simulink model "NGGenset_Test_System"  (Simulink 8.1)
settings: Solver=ode3  SolverMode=SingleTasking  StartTime=0.0  StopTime=150  FixedStep=Ts  RelTol=1e-3
PostLoadFcn:
  | Ts=50e-6;
InitFcn:
  | Ts=50e-6;
undefined symbols (not defined in the file): another_event_name, DiscIntNeverNeededParam, fdesignblkfcn, gcbh, Gen_900kW_external_control, HIL_GenSet, Left, my_event_name, ph, type, V
libraries: powerlib x47, simulink x40, powerlib_extras x28, rtio_opalrt_common x21, dspsigops x7, breakers_1ph_3ph x7, rtio_generic_modbus x7, simulink_extras x6, cables_lib x5, rteventslib x4, rtlab x3, discretizing x2
(part 4 of 5)

== system NGGenset_Test_System/SM_Master/Generator/Woodward Outputs/TSDIO - Gr3 ==
  TSDout : Inport
  Bus Creator : BusCreator  Inputs=16
  Bus Creator1 : BusCreator  Inputs=16
  Bus Creator2 : BusCreator  Inputs=2
  Bus Selector : BusSelector  OutputSignals=16 TSDOUT GR3.states.CH16-23.states 17,16 TSDOUT GR3.times CH16-23.times17,16 TSDOUT GR3.states.CH16-23.states 18,16 TSDOUT GR3.times CH16-23.times18,16 TSDOUT GR3.states.CH16-23.states 19,16 TSDOUT GR3.times CH16-23.times19,16 TSDOUT GR3.states.CH16-23.states 20,16 TSDOUT GR3.times CH16-23.times20,16 TSDOUT GR3.states.CH16-23.states 21,16 TSDOUT GR3.times CH16-23.times21,16 TSDOUT GR3.states.CH16-23.states 22,16 TSDOUT GR3.times CH16-23.times22,16 TSDOUT GR3.states.CH16-23.states 23,16 TSDOUT GR3.times CH16-23.times23,16 TSDOUT GR3.states.CH16-23.states 24,16 TSDOUT GR3.times CH16-23.times24
  Bus Selector1 : BusSelector  OutputSignals=16 TSDOUT GR3.states.CH24-31.states 25,16 TSDOUT GR3.times CH24-31.times25,16 TSDOUT GR3.states.CH24-31.states 26,16 TSDOUT GR3.times CH24-31.times26,16 TSDOUT GR3.states.CH24-31.states 27,16 TSDOUT GR3.times CH24-31.times27,16 TSDOUT GR3.states.CH24-31.states 28,16 TSDOUT GR3.times CH24-31.times28,16 TSDOUT GR3.states.CH24-31.states 29,16 TSDOUT GR3.times CH24-31.times29,16 TSDOUT GR3.states.CH24-31.states 30,16 TSDOUT GR3.times CH24-31.times30,16 TSDOUT GR3.states.CH24-31.states 31,16 TSDOUT GR3.times CH24-31.times31,16 TSDOUT GR3.states.CH24-31.states 32,16 TSDOUT GR3.times CH24-31.times32
  EventDetector : rtio_opalrt_common/EventDetector  CtrlName='OpCtrl'  portNb=7  FcnNos=Slot 3 Module A Subsection 3  size=32  maxcount=8  nbChannels=8  width=4  timeUnit=Time ratio  sampleTime=0  numwidth=4
      settings: AttributesFormatString=%<CtrlName>
  EventDetector1 : rtio_opalrt_common/EventDetector  CtrlName='OpCtrl'  portNb=8  FcnNos=Slot 3 Module A Subsection 4  size=32  maxcount=8  nbChannels=8  width=4  timeUnit=Time ratio  sampleTime=0  numwidth=4
      settings: AttributesFormatString=%<CtrlName>
  EventGenerator : rtio_opalrt_common/EventGenerator  CtrlName='OpCtrl'  portNb=7  FcnNos=Slot 3 Module B Subsection 3  size=32  count=8  nbChannels=8  width=4  timeUnit=Time ratio  numwidth=4
      settings: AttributesFormatString=%<CtrlName>
  EventGenerator1 : rtio_opalrt_common/EventGenerator  CtrlName='OpCtrl'  portNb=8  FcnNos=Slot 3 Module B Subsection 4  size=32  count=8  nbChannels=8  width=4  timeUnit=Time ratio  numwidth=4
      settings: AttributesFormatString=%<CtrlName>
  Terminator{,1..3} (4 alike) : Terminator
  TSDin : Outport
  wires:
  TSDout/1 -> Bus Selector/1, Bus Selector1/1
  Bus Selector/16 -> EventGenerator/16  "<times24>"
  Bus Selector/15 -> EventGenerator/15  "<states 24>"
  Bus Selector/14 -> EventGenerator/14  "<times23>"
  Bus Selector/13 -> EventGenerator/13  "<states 23>"
  Bus Selector/12 -> EventGenerator/12  "<times22>"
  Bus Selector/11 -> EventGenerator/11  "<states 22>"
  Bus Selector/10 -> EventGenerator/10  "<times21>"
  Bus Selector/9 -> EventGenerator/9  "<states 21>"
  Bus Selector/8 -> EventGenerator/8  "<times20>"
  Bus Selector/7 -> EventGenerator/7  "<states 20>"
  Bus Selector/6 -> EventGenerator/6  "<times19>"
  Bus Selector/5 -> EventGenerator/5  "<states 19>"
  Bus Selector/4 -> EventGenerator/4  "<times18>"
  Bus Selector/3 -> EventGenerator/3  "<states 18>"
  Bus Selector/2 -> EventGenerator/2  "<times17>"
  Bus Selector/1 -> EventGenerator/1  "<states 17>"
  EventGenerator/1 -> Terminator/1
  EventDetector/16 -> Bus Creator/16  "times8"
  EventDetector/15 -> Bus Creator/15  "states8"
  EventDetector/14 -> Bus Creator/14  "times7"
  EventDetector/13 -> Bus Creator/13  "states7"
  EventDetector/12 -> Bus Creator/12  "times6"
  EventDetector/11 -> Bus Creator/11  "states6"
  EventDetector/10 -> Bus Creator/10  "times5"
  EventDetector/9 -> Bus Creator/9  "states5"
  EventDetector/8 -> Bus Creator/8  "times4"
  EventDetector/7 -> Bus Creator/7  "states4"
  EventDetector/6 -> Bus Creator/6  "times3"
  EventDetector/5 -> Bus Creator/5  "states3"
  EventDetector/4 -> Bus Creator/4  "times2"
  EventDetector/3 -> Bus Creator/3  "states2"
  EventDetector/2 -> Bus Creator/2  "times1"
  EventDetector/1 -> Bus Creator/1  "states1"
  EventDetector/17 -> Terminator1/1
  EventGenerator1/1 -> Terminator2/1
  Bus Selector1/1 -> EventGenerator1/1  "<states 25>"
  Bus Selector1/2 -> EventGenerator1/2  "<times25>"
  Bus Selector1/3 -> EventGenerator1/3  "<states 26>"
  Bus Selector1/4 -> EventGenerator1/4  "<times26>"
  Bus Selector1/5 -> EventGenerator1/5  "<states 27>"
  Bus Selector1/6 -> EventGenerator1/6  "<times27>"
  Bus Selector1/7 -> EventGenerator1/7  "<states 28>"
  Bus Selector1/8 -> EventGenerator1/8  "<times28>"
  Bus Selector1/9 -> EventGenerator1/9  "<states 29>"
  Bus Selector1/10 -> EventGenerator1/10  "<times29>"
  Bus Selector1/11 -> EventGenerator1/11  "<states 30>"
  Bus Selector1/12 -> EventGenerator1/12  "<times30>"
  Bus Selector1/13 -> EventGenerator1/13  "<states 31>"
  Bus Selector1/14 -> EventGenerator1/14  "<times31>"
  Bus Selector1/15 -> EventGenerator1/15  "<states 32>"
  Bus Selector1/16 -> EventGenerator1/16  "<times32>"
  Bus Creator1/1 -> Bus Creator2/2  "CH24-31"
  EventDetector1/16 -> Bus Creator1/16  "times6"
  EventDetector1/15 -> Bus Creator1/15  "states6"
  EventDetector1/14 -> Bus Creator1/14  "times5"
  EventDetector1/13 -> Bus Creator1/13  "states5"
  EventDetector1/12 -> Bus Creator1/12  "times4"
  EventDetector1/11 -> Bus Creator1/11  "states4"
  EventDetector1/10 -> Bus Creator1/10  "times3"
  EventDetector1/9 -> Bus Creator1/9  "states3"
  EventDetector1/8 -> Bus Creator1/8  "times2"
  EventDetector1/7 -> Bus Creator1/7  "states2"
  EventDetector1/6 -> Bus Creator1/6  "times1"
  EventDetector1/5 -> Bus Creator1/5  "states1"
  EventDetector1/4 -> Bus Creator1/4  "times2"
  EventDetector1/3 -> Bus Creator1/3  "states2"
  EventDetector1/2 -> Bus Creator1/2  "times1"
  EventDetector1/1 -> Bus Creator1/1  "states1"
  EventDetector1/17 -> Terminator3/1  "states7"
  Bus Creator/1 -> Bus Creator2/1  "CH16-23"
  Bus Creator2/1 -> TSDin/1  "TSDIN"

== system NGGenset_Test_System/SM_Master/Generator/Woodward Outputs/Woodward Primary Inputs ==
  Bias-ctrl : Inport
  Bus Creator : BusCreator
  Bus Creator1 : BusCreator
  Constant{,5,10..11} (4 alike) : Constant  Value=1.00
  Constant{1,3..4,6,8..9} (6 alike) : Constant  Value=0
  Constant2 : Constant  Value=20
  Constant7 : Constant  Value=20
  Demux1 : Demux  Outputs=16
  Divide{,1..3} (4 alike) : Product  Inputs=*/
  GR1 B AIN (CH00-15) : Subsystem
  Lowpass Filter : Subsystem  DialogController=fdesignblkfcn  DialogControllerArgs=DataTag4  InitFcn=fdesignblkfcn(gcbh, {'InitFcn'});  mask(Lowpass Filter){}
      mask help: Design a lowpass filter
      settings: CopyFcn=fdesignblkfcn(gcbh, {'CopyFcn'});
      mask Help: helpview(mapfilelocation('dsp'), 'dsplowpassfilter');
      mask Display: disp('Lowpass')
  Lowpass Filter1 : Subsystem  DialogController=fdesignblkfcn  DialogControllerArgs=DataTag6  InitFcn=fdesignblkfcn(gcbh, {'InitFcn'});  mask(Lowpass Filter){}
      mask help: Design a lowpass filter
      settings: CopyFcn=fdesignblkfcn(gcbh, {'CopyFcn'});
      mask Help: helpview(mapfilelocation('dsp'), 'dsplowpassfilter');
      mask Display: disp('Lowpass')
  Lowpass Filter2 : Subsystem  DialogController=fdesignblkfcn  DialogControllerArgs=DataTag8  InitFcn=fdesignblkfcn(gcbh, {'InitFcn'});  mask(Lowpass Filter){}
      mask help: Design a lowpass filter
      settings: CopyFcn=fdesignblkfcn(gcbh, {'CopyFcn'});
      mask Help: helpview(mapfilelocation('dsp'), 'dsplowpassfilter');
      mask Display: disp('Lowpass')
  Lowpass Filter3 : Subsystem  DialogController=fdesignblkfcn  DialogControllerArgs=DataTag10  InitFcn=fdesignblkfcn(gcbh, {'InitFcn'});  mask(Lowpass Filter){}
      mask help: Design a lowpass filter
      settings: CopyFcn=fdesignblkfcn(gcbh, {'CopyFcn'});
      mask Help: helpview(mapfilelocation('dsp'), 'dsplowpassfilter');
      mask Display: disp('Lowpass')
  Sum{,1..3} (4 alike) : Sum  Inputs=|+-
  Switch{,1..3} (4 alike) : Switch  Threshold=0.5
  Gen1 Gov and AVR : Outport
  Gen2 Gov and AVR : Outport  Port=2
  wires:
  GR1 B AIN (CH00-15)/1(Out1) -> [AINs_Gr1], Demux1/1
  Demux1/1 -> Divide/1
  Demux1/2 -> Divide1/1
  Constant2/1 -> Divide1/2, Divide/2
  Divide/1 -> Sum/1
  Divide1/1 -> Sum1/1
  Constant3/1 -> Sum/2
  Constant4/1 -> Sum1/2
  Sum/1 -> Lowpass Filter/1(In)
  Switch/1 -> Bus Creator/3  "Gen1 Gov"
  Switch1/1 -> Bus Creator/4  "Gen1 AVR"
  Sum1/1 -> Lowpass Filter1/1(In)
  Constant1/1 -> Switch/3, Switch1/3
  Bias-ctrl/1 -> Switch/2, Switch1/2, Switch2/2, Switch3/2
  Lowpass Filter/1(Out) -> Switch/1
  Lowpass Filter1/1(Out) -> Switch1/1
  Constant5/1 -> Bus Creator/2  "Gen1 Ref AVR"
  Constant/1 -> Bus Creator/1  "Gen1 Ref GOV"
  Demux1/3 -> Divide2/1
  Demux1/4 -> Divide3/1
  Constant7/1 -> Divide3/2, Divide2/2
  Divide2/1 -> Sum2/1
  Divide3/1 -> Sum3/1
  Constant8/1 -> Sum2/2
  Constant9/1 -> Sum3/2
  Sum2/1 -> Lowpass Filter2/1(In)
  Switch2/1 -> Bus Creator1/3  "Gen2 GOV"
  Switch3/1 -> Bus Creator1/4  "Gen2 AVR"
  Sum3/1 -> Lowpass Filter3/1(In)
  Constant6/1 -> Switch2/3, Switch3/3
  Lowpass Filter2/1(Out) -> Switch2/1
  Lowpass Filter3/1(Out) -> Switch3/1
  Constant11/1 -> Bus Creator1/2  "Gen2 Ref AVR"
  Constant10/1 -> Bus Creator1/1  "Gen2 Ref GOV"
  Bus Creator/1 -> Gen1 Gov and AVR/1
  Bus Creator1/1 -> Gen2 Gov and AVR/1

== system NGGenset_Test_System/SM_Master/MODBUS1/SEL_787_Relay/PQ_Calculator ==
  Vabc : Inport
  Iabc : Inport  Port=2
  3-phase  Instantaneous  Active & Reactive Power : powerlib_extras/Measurements/3-phase  Instantaneous  Active & Reactive Power
  Demux : Demux  Outputs=2
  Discrete  Mean value2 : powerlib_extras/Discrete Measurements/Discrete  Mean value  Freq=60  Vinit=0  Ts=Ts
  P : Outport
  Q : Outport  Port=2
  wires:
  3-phase  Instantaneous  Active & Reactive Power/1 -> Discrete  Mean value2/1
  Discrete  Mean value2/1 -> Demux/1
  Vabc/1 -> 3-phase  Instantaneous  Active & Reactive Power/1
  Iabc/1 -> 3-phase  Instantaneous  Active & Reactive Power/2
  Demux/1 -> P/1  "P"
  Demux/2 -> Q/1  "Q"

== system NGGenset_Test_System/SM_Master/MODBUS1/SEL_787_Relay/RMS_Calculator ==
  Signal : Inport
  Discrete  Mean value6 : powerlib_extras/Discrete Measurements/Discrete  Mean value  Freq=60  Vinit=0  Ts=Ts
  Product3 : Product  RndMeth=Zero
  Signed Sqrt : Sqrt  SaturateOnIntegerOverflow=on
  RMS_Signal : Outport
  wires:
  Signal/1 -> Product3/1, Product3/2
  Product3/1 -> Discrete  Mean value6/1
  Discrete  Mean value6/1 -> Signed Sqrt/1
  Signed Sqrt/1 -> RMS_Signal/1

== system NGGenset_Test_System/SM_Master/MODBUS1/SEL_787_Relay/RMS_Calculator1 ==
  Signal : Inport
  Discrete  Mean value6 : powerlib_extras/Discrete Measurements/Discrete  Mean value  Freq=60  Vinit=0  Ts=Ts
  Product3 : Product  RndMeth=Zero
  Signed Sqrt : Sqrt  SaturateOnIntegerOverflow=on
  RMS_Signal : Outport
  wires:
  Signal/1 -> Product3/1, Product3/2
  Product3/1 -> Discrete  Mean value6/1
  Discrete  Mean value6/1 -> Signed Sqrt/1
  Signed Sqrt/1 -> RMS_Signal/1

== system NGGenset_Test_System/SM_Master/MODBUS1/SEL_787_Relay/pf_Calculator ==
  P : Inport
  Q : Inport  Port=2
  Fcn : Fcn  Expr=u(1) / sqrt(u(1)^2 + u(2)^2)
  Fcn1 : Fcn  Expr=sqrt(u(1)^2 + u(2)^2)
  Mux : Mux  Inputs=2
  Mux1 : Mux  Inputs=2
  Scope : Scope
      settings: YMin=0.8475  YMax=0.875  SaveName=ScopeData2
  pf : Outport
  S : Outport  Port=2
  wires:
  Fcn1/1 -> S/1
  Mux1/1 -> Fcn1/1
  Fcn/1 -> Scope/1, pf/1
  Mux/1 -> Fcn/1
  P/1 -> Mux1/1, Mux/1
  Q/1 -> Mux1/2, Mux/2

== system NGGenset_Test_System/SM_Master/MODBUS10/SEL_787_Relay/PQ_Calculator ==
  Vabc : Inport
  Iabc : Inport  Port=2
  3-phase  Instantaneous  Active & Reactive Power : powerlib_extras/Measurements/3-phase  Instantaneous  Active & Reactive Power
  Demux : Demux  Outputs=2
  Discrete  Mean value2 : powerlib_extras/Discrete Measurements/Discrete  Mean value  Freq=60  Vinit=0  Ts=Ts
  P : Outport
  Q : Outport  Port=2
  wires:
  3-phase  Instantaneous  Active & Reactive Power/1 -> Discrete  Mean value2/1
  Discrete  Mean value2/1 -> Demux/1
  Vabc/1 -> 3-phase  Instantaneous  Active & Reactive Power/1
  Iabc/1 -> 3-phase  Instantaneous  Active & Reactive Power/2
  Demux/1 -> P/1  "P"
  Demux/2 -> Q/1  "Q"

== system NGGenset_Test_System/SM_Master/MODBUS10/SEL_787_Relay/RMS_Calculator ==
  Signal : Inport
  Discrete  Mean value6 : powerlib_extras/Discrete Measurements/Discrete  Mean value  Freq=60  Vinit=0  Ts=Ts
  Product3 : Product  RndMeth=Zero
  Signed Sqrt : Sqrt  SaturateOnIntegerOverflow=on
  RMS_Signal : Outport
  wires:
  Signal/1 -> Product3/1, Product3/2
  Product3/1 -> Discrete  Mean value6/1
  Discrete  Mean value6/1 -> Signed Sqrt/1
  Signed Sqrt/1 -> RMS_Signal/1

== system NGGenset_Test_System/SM_Master/MODBUS10/SEL_787_Relay/RMS_Calculator1 ==
  Signal : Inport
  Discrete  Mean value6 : powerlib_extras/Discrete Measurements/Discrete  Mean value  Freq=60  Vinit=0  Ts=Ts
  Product3 : Product  RndMeth=Zero
  Signed Sqrt : Sqrt  SaturateOnIntegerOverflow=on
  RMS_Signal : Outport
  wires:
  Signal/1 -> Product3/1, Product3/2
  Product3/1 -> Discrete  Mean value6/1
  Discrete  Mean value6/1 -> Signed Sqrt/1
  Signed Sqrt/1 -> RMS_Signal/1

== system NGGenset_Test_System/SM_Master/MODBUS10/SEL_787_Relay/pf_Calculator ==
  P : Inport
  Q : Inport  Port=2
  Fcn : Fcn  Expr=u(1) / sqrt(u(1)^2 + u(2)^2)
  Fcn1 : Fcn  Expr=sqrt(u(1)^2 + u(2)^2)
  Mux : Mux  Inputs=2
  Mux1 : Mux  Inputs=2
  Scope : Scope
      settings: YMin=0.8475  YMax=0.875  SaveName=ScopeData2
  pf : Outport
  S : Outport  Port=2
  wires:
  Fcn1/1 -> S/1
  Mux1/1 -> Fcn1/1
  Fcn/1 -> Scope/1, pf/1
  Mux/1 -> Fcn/1
  P/1 -> Mux1/1, Mux/1
  Q/1 -> Mux1/2, Mux/2

== system NGGenset_Test_System/SM_Master/MODBUS2/SEL_787_Relay/PQ_Calculator ==
  Vabc : Inport
  Iabc : Inport  Port=2
  3-phase  Instantaneous  Active & Reactive Power : powerlib_extras/Measurements/3-phase  Instantaneous  Active & Reactive Power
  Demux : Demux  Outputs=2
  Discrete  Mean value2 : powerlib_extras/Discrete Measurements/Discrete  Mean value  Freq=60  Vinit=0  Ts=Ts
  P : Outport
  Q : Outport  Port=2
  wires:
  3-phase  Instantaneous  Active & Reactive Power/1 -> Discrete  Mean value2/1
  Discrete  Mean value2/1 -> Demux/1
  Vabc/1 -> 3-phase  Instantaneous  Active & Reactive Power/1
  Iabc/1 -> 3-phase  Instantaneous  Active & Reactive Power/2
  Demux/1 -> P/1  "P"
  Demux/2 -> Q/1  "Q"

== system NGGenset_Test_System/SM_Master/MODBUS2/SEL_787_Relay/RMS_Calculator ==
  Signal : Inport
  Discrete  Mean value6 : powerlib_extras/Discrete Measurements/Discrete  Mean value  Freq=60  Vinit=0  Ts=Ts
  Product3 : Product  RndMeth=Zero
  Signed Sqrt : Sqrt  SaturateOnIntegerOverflow=on
  RMS_Signal : Outport
  wires:
  Signal/1 -> Product3/1, Product3/2
  Product3/1 -> Discrete  Mean value6/1
  Discrete  Mean value6/1 -> Signed Sqrt/1
  Signed Sqrt/1 -> RMS_Signal/1

== system NGGenset_Test_System/SM_Master/MODBUS2/SEL_787_Relay/RMS_Calculator1 ==
  Signal : Inport
  Discrete  Mean value6 : powerlib_extras/Discrete Measurements/Discrete  Mean value  Freq=60  Vinit=0  Ts=Ts
  Product3 : Product  RndMeth=Zero
  Signed Sqrt : Sqrt  SaturateOnIntegerOverflow=on
  RMS_Signal : Outport
  wires:
  Signal/1 -> Product3/1, Product3/2
  Product3/1 -> Discrete  Mean value6/1
  Discrete  Mean value6/1 -> Signed Sqrt/1
  Signed Sqrt/1 -> RMS_Signal/1

== system NGGenset_Test_System/SM_Master/MODBUS2/SEL_787_Relay/pf_Calculator ==
  P : Inport
  Q : Inport  Port=2
  Fcn : Fcn  Expr=u(1) / sqrt(u(1)^2 + u(2)^2)
  Fcn1 : Fcn  Expr=sqrt(u(1)^2 + u(2)^2)
  Mux : Mux  Inputs=2
  Mux1 : Mux  Inputs=2
  Scope : Scope
      settings: YMin=0.8475  YMax=0.875  SaveName=ScopeData2
  pf : Outport
  S : Outport  Port=2
  wires:
  Fcn1/1 -> S/1
  Mux1/1 -> Fcn1/1
  Fcn/1 -> Scope/1, pf/1
  Mux/1 -> Fcn/1
  P/1 -> Mux1/1, Mux/1
  Q/1 -> Mux1/2, Mux/2

== system NGGenset_Test_System/SM_Master/MODBUS4/SEL_787_Relay/PQ_Calculator ==
  Vabc : Inport
  Iabc : Inport  Port=2
  3-phase  Instantaneous  Active & Reactive Power : powerlib_extras/Measurements/3-phase  Instantaneous  Active & Reactive Power
  Demux : Demux  Outputs=2
  Discrete  Mean value2 : powerlib_extras/Discrete Measurements/Discrete  Mean value  Freq=60  Vinit=0  Ts=Ts
  P : Outport
  Q : Outport  Port=2
  wires:
  3-phase  Instantaneous  Active & Reactive Power/1 -> Discrete  Mean value2/1
  Discrete  Mean value2/1 -> Demux/1
  Vabc/1 -> 3-phase  Instantaneous  Active & Reactive Power/1
  Iabc/1 -> 3-phase  Instantaneous  Active & Reactive Power/2
  Demux/1 -> P/1  "P"
  Demux/2 -> Q/1  "Q"

== system NGGenset_Test_System/SM_Master/MODBUS4/SEL_787_Relay/RMS_Calculator ==
  Signal : Inport
  Discrete  Mean value6 : powerlib_extras/Discrete Measurements/Discrete  Mean value  Freq=60  Vinit=0  Ts=Ts
  Product3 : Product  RndMeth=Zero
  Signed Sqrt : Sqrt  SaturateOnIntegerOverflow=on
  RMS_Signal : Outport
  wires:
  Signal/1 -> Product3/1, Product3/2
  Product3/1 -> Discrete  Mean value6/1
  Discrete  Mean value6/1 -> Signed Sqrt/1
  Signed Sqrt/1 -> RMS_Signal/1

== system NGGenset_Test_System/SM_Master/MODBUS4/SEL_787_Relay/RMS_Calculator1 ==
  Signal : Inport
  Discrete  Mean value6 : powerlib_extras/Discrete Measurements/Discrete  Mean value  Freq=60  Vinit=0  Ts=Ts
  Product3 : Product  RndMeth=Zero
  Signed Sqrt : Sqrt  SaturateOnIntegerOverflow=on
  RMS_Signal : Outport
  wires:
  Signal/1 -> Product3/1, Product3/2
  Product3/1 -> Discrete  Mean value6/1
  Discrete  Mean value6/1 -> Signed Sqrt/1
  Signed Sqrt/1 -> RMS_Signal/1

== system NGGenset_Test_System/SM_Master/MODBUS4/SEL_787_Relay/pf_Calculator ==
  P : Inport
  Q : Inport  Port=2
  Fcn : Fcn  Expr=u(1) / sqrt(u(1)^2 + u(2)^2)
  Fcn1 : Fcn  Expr=sqrt(u(1)^2 + u(2)^2)
  Mux : Mux  Inputs=2
  Mux1 : Mux  Inputs=2
  Scope : Scope
      settings: YMin=0.8475  YMax=0.875  SaveName=ScopeData2
  pf : Outport
  S : Outport  Port=2
  wires:
  Fcn1/1 -> S/1
  Mux1/1 -> Fcn1/1
  Fcn/1 -> Scope/1, pf/1
  Mux/1 -> Fcn/1
  P/1 -> Mux1/1, Mux/1
  Q/1 -> Mux1/2, Mux/2

== system NGGenset_Test_System/SM_Master/MODBUS5/SEL_787_Relay/PQ_Calculator ==
  Vabc : Inport
  Iabc : Inport  Port=2
  3-phase  Instantaneous  Active & Reactive Power : powerlib_extras/Measurements/3-phase  Instantaneous  Active & Reactive Power
  Demux : Demux  Outputs=2
  Discrete  Mean value2 : powerlib_extras/Discrete Measurements/Discrete  Mean value  Freq=60  Vinit=0  Ts=Ts
  P : Outport
  Q : Outport  Port=2
  wires:
  3-phase  Instantaneous  Active & Reactive Power/1 -> Discrete  Mean value2/1
  Discrete  Mean value2/1 -> Demux/1
  Vabc/1 -> 3-phase  Instantaneous  Active & Reactive Power/1
  Iabc/1 -> 3-phase  Instantaneous  Active & Reactive Power/2
  Demux/1 -> P/1  "P"
  Demux/2 -> Q/1  "Q"

== system NGGenset_Test_System/SM_Master/MODBUS5/SEL_787_Relay/RMS_Calculator ==
  Signal : Inport
  Discrete  Mean value6 : powerlib_extras/Discrete Measurements/Discrete  Mean value  Freq=60  Vinit=0  Ts=Ts
  Product3 : Product  RndMeth=Zero
  Signed Sqrt : Sqrt  SaturateOnIntegerOverflow=on
  RMS_Signal : Outport
  wires:
  Signal/1 -> Product3/1, Product3/2
  Product3/1 -> Discrete  Mean value6/1
  Discrete  Mean value6/1 -> Signed Sqrt/1
  Signed Sqrt/1 -> RMS_Signal/1

== system NGGenset_Test_System/SM_Master/MODBUS5/SEL_787_Relay/RMS_Calculator1 ==
  Signal : Inport
  Discrete  Mean value6 : powerlib_extras/Discrete Measurements/Discrete  Mean value  Freq=60  Vinit=0  Ts=Ts
  Product3 : Product  RndMeth=Zero
  Signed Sqrt : Sqrt  SaturateOnIntegerOverflow=on
  RMS_Signal : Outport
  wires:
  Signal/1 -> Product3/1, Product3/2
  Product3/1 -> Discrete  Mean value6/1
  Discrete  Mean value6/1 -> Signed Sqrt/1
  Signed Sqrt/1 -> RMS_Signal/1

== system NGGenset_Test_System/SM_Master/MODBUS5/SEL_787_Relay/pf_Calculator ==
  P : Inport
  Q : Inport  Port=2
  Fcn : Fcn  Expr=u(1) / sqrt(u(1)^2 + u(2)^2)
  Fcn1 : Fcn  Expr=sqrt(u(1)^2 + u(2)^2)
  Mux : Mux  Inputs=2
  Mux1 : Mux  Inputs=2
  Scope : Scope
      settings: YMin=0.8475  YMax=0.875  SaveName=ScopeData2
  pf : Outport
  S : Outport  Port=2
  wires:
  Fcn1/1 -> S/1
  Mux1/1 -> Fcn1/1
  Fcn/1 -> Scope/1, pf/1
  Mux/1 -> Fcn/1
  P/1 -> Mux1/1, Mux/1
  Q/1 -> Mux1/2, Mux/2

== system NGGenset_Test_System/SM_Master/MODBUS6/SEL_787_Relay/PQ_Calculator ==
  Vabc : Inport
  Iabc : Inport  Port=2
  3-phase  Instantaneous  Active & Reactive Power : powerlib_extras/Measurements/3-phase  Instantaneous  Active & Reactive Power
  Demux : Demux  Outputs=2
  Discrete  Mean value2 : powerlib_extras/Discrete Measurements/Discrete  Mean value  Freq=60  Vinit=0  Ts=Ts
  P : Outport
  Q : Outport  Port=2
  wires:
  3-phase  Instantaneous  Active & Reactive Power/1 -> Discrete  Mean value2/1
  Discrete  Mean value2/1 -> Demux/1
  Vabc/1 -> 3-phase  Instantaneous  Active & Reactive Power/1
  Iabc/1 -> 3-phase  Instantaneous  Active & Reactive Power/2
  Demux/1 -> P/1  "P"
  Demux/2 -> Q/1  "Q"

== system NGGenset_Test_System/SM_Master/MODBUS6/SEL_787_Relay/RMS_Calculator ==
  Signal : Inport
  Discrete  Mean value6 : powerlib_extras/Discrete Measurements/Discrete  Mean value  Freq=60  Vinit=0  Ts=Ts
  Product3 : Product  RndMeth=Zero
  Signed Sqrt : Sqrt  SaturateOnIntegerOverflow=on
  RMS_Signal : Outport
  wires:
  Signal/1 -> Product3/1, Product3/2
  Product3/1 -> Discrete  Mean value6/1
  Discrete  Mean value6/1 -> Signed Sqrt/1
  Signed Sqrt/1 -> RMS_Signal/1

== system NGGenset_Test_System/SM_Master/MODBUS6/SEL_787_Relay/RMS_Calculator1 ==
  Signal : Inport
  Discrete  Mean value6 : powerlib_extras/Discrete Measurements/Discrete  Mean value  Freq=60  Vinit=0  Ts=Ts
  Product3 : Product  RndMeth=Zero
  Signed Sqrt : Sqrt  SaturateOnIntegerOverflow=on
  RMS_Signal : Outport
  wires:
  Signal/1 -> Product3/1, Product3/2
  Product3/1 -> Discrete  Mean value6/1
  Discrete  Mean value6/1 -> Signed Sqrt/1
  Signed Sqrt/1 -> RMS_Signal/1

== system NGGenset_Test_System/SM_Master/MODBUS6/SEL_787_Relay/pf_Calculator ==
  P : Inport
  Q : Inport  Port=2
  Fcn : Fcn  Expr=u(1) / sqrt(u(1)^2 + u(2)^2)
  Fcn1 : Fcn  Expr=sqrt(u(1)^2 + u(2)^2)
  Mux : Mux  Inputs=2
  Mux1 : Mux  Inputs=2
  Scope : Scope
      settings: YMin=0.8475  YMax=0.875  SaveName=ScopeData2
  pf : Outport
  S : Outport  Port=2
  wires:
  Fcn1/1 -> S/1
  Mux1/1 -> Fcn1/1
  Fcn/1 -> Scope/1, pf/1
  Mux/1 -> Fcn/1
  P/1 -> Mux1/1, Mux/1
  Q/1 -> Mux1/2, Mux/2

== system NGGenset_Test_System/SM_Master/MODBUS8/SEL_787_Relay/PQ_Calculator ==
  Vabc : Inport
  Iabc : Inport  Port=2
  3-phase  Instantaneous  Active & Reactive Power : powerlib_extras/Measurements/3-phase  Instantaneous  Active & Reactive Power
  Demux : Demux  Outputs=2
  Discrete  Mean value2 : powerlib_extras/Discrete Measurements/Discrete  Mean value  Freq=60  Vinit=0  Ts=Ts
  P : Outport
  Q : Outport  Port=2
  wires:
  3-phase  Instantaneous  Active & Reactive Power/1 -> Discrete  Mean value2/1
  Discrete  Mean value2/1 -> Demux/1
  Vabc/1 -> 3-phase  Instantaneous  Active & Reactive Power/1
  Iabc/1 -> 3-phase  Instantaneous  Active & Reactive Power/2
  Demux/1 -> P/1  "P"
  Demux/2 -> Q/1  "Q"

== system NGGenset_Test_System/SM_Master/MODBUS8/SEL_787_Relay/RMS_Calculator ==
  Signal : Inport
  Discrete  Mean value6 : powerlib_extras/Discrete Measurements/Discrete  Mean value  Freq=60  Vinit=0  Ts=Ts
  Product3 : Product  RndMeth=Zero
  Signed Sqrt : Sqrt  SaturateOnIntegerOverflow=on
  RMS_Signal : Outport
  wires:
  Signal/1 -> Product3/1, Product3/2
  Product3/1 -> Discrete  Mean value6/1
  Discrete  Mean value6/1 -> Signed Sqrt/1
  Signed Sqrt/1 -> RMS_Signal/1

== system NGGenset_Test_System/SM_Master/MODBUS8/SEL_787_Relay/RMS_Calculator1 ==
  Signal : Inport
  Discrete  Mean value6 : powerlib_extras/Discrete Measurements/Discrete  Mean value  Freq=60  Vinit=0  Ts=Ts
  Product3 : Product  RndMeth=Zero
  Signed Sqrt : Sqrt  SaturateOnIntegerOverflow=on
  RMS_Signal : Outport
  wires:
  Signal/1 -> Product3/1, Product3/2
  Product3/1 -> Discrete  Mean value6/1
  Discrete  Mean value6/1 -> Signed Sqrt/1
  Signed Sqrt/1 -> RMS_Signal/1

== system NGGenset_Test_System/SM_Master/MODBUS8/SEL_787_Relay/pf_Calculator ==
  P : Inport
  Q : Inport  Port=2
  Fcn : Fcn  Expr=u(1) / sqrt(u(1)^2 + u(2)^2)
  Fcn1 : Fcn  Expr=sqrt(u(1)^2 + u(2)^2)
  Mux : Mux  Inputs=2
  Mux1 : Mux  Inputs=2
  Scope : Scope
      settings: YMin=0.8475  YMax=0.875  SaveName=ScopeData2
  pf : Outport
  S : Outport  Port=2
  wires:
  Fcn1/1 -> S/1
  Mux1/1 -> Fcn1/1
  Fcn/1 -> Scope/1, pf/1
  Mux/1 -> Fcn/1
  P/1 -> Mux1/1, Mux/1
  Q/1 -> Mux1/2, Mux/2

== system NGGenset_Test_System/SC_Console/Woodward/16TSDIn/16 TSDOut GR3/Dout state ctrl/Dout_CH16_CH23 ==
  Bus Creator1 : BusCreator  Inputs=8
  Dout_CH{16..23} (8 alike) : Constant  Value=[1 0 1 0]
  Manual Switch{17..24} (8 alike) : ManualSwitch
  Zero_Dout_CH{16..23} (8 alike) : Constant  Value=[0 0 0 0]
  Dout_CH8_CH15 : Outport
  wires:
  Manual Switch24/1 -> Bus Creator1/8  "states 24"
  Manual Switch23/1 -> Bus Creator1/7  "states 23"
  Manual Switch22/1 -> Bus Creator1/6  "states 22"
  Manual Switch21/1 -> Bus Creator1/5  "states 21"
  Manual Switch20/1 -> Bus Creator1/4  "states 20"
  Manual Switch19/1 -> Bus Creator1/3  "states 19"
  Manual Switch18/1 -> Bus Creator1/2  "states 18"
  Manual Switch17/1 -> Bus Creator1/1  "states 17"
  Zero_Dout_CH23/1 -> Manual Switch24/2
  Dout_CH23/1 -> Manual Switch24/1
  Zero_Dout_CH22/1 -> Manual Switch23/2
  Dout_CH22/1 -> Manual Switch23/1
  Zero_Dout_CH21/1 -> Manual Switch22/2
  Dout_CH21/1 -> Manual Switch22/1
  Zero_Dout_CH20/1 -> Manual Switch21/2
  Dout_CH20/1 -> Manual Switch21/1
  Zero_Dout_CH19/1 -> Manual Switch20/2
  Dout_CH19/1 -> Manual Switch20/1
  Zero_Dout_CH18/1 -> Manual Switch19/2
  Dout_CH18/1 -> Manual Switch19/1
  Zero_Dout_CH17/1 -> Manual Switch18/2
  Dout_CH17/1 -> Manual Switch18/1
  Zero_Dout_CH16/1 -> Manual Switch17/2
  Dout_CH16/1 -> Manual Switch17/1
  Bus Creator1/1 -> Dout_CH8_CH15/1

== system NGGenset_Test_System/SC_Console/Woodward/16TSDIn/16 TSDOut GR3/Dout state ctrl/Dout_CH24_CH31 ==
  Bus Creator : BusCreator  Inputs=8
  Dout_CH{24..31} (8 alike) : Constant  Value=[1 0 1 0]
  Manual Switch{25..32} (8 alike) : ManualSwitch
  Zero_Dout_CH{24..31} (8 alike) : Constant  Value=[0 0 0 0]
  Dout_CH8_CH15 : Outport
  wires:
  Bus Creator/1 -> Dout_CH8_CH15/1
  Dout_CH24/1 -> Manual Switch25/1
  Zero_Dout_CH24/1 -> Manual Switch25/2
  Dout_CH25/1 -> Manual Switch26/1
  Zero_Dout_CH25/1 -> Manual Switch26/2
  Dout_CH26/1 -> Manual Switch27/1
  Zero_Dout_CH26/1 -> Manual Switch27/2
  Dout_CH27/1 -> Manual Switch28/1
  Zero_Dout_CH27/1 -> Manual Switch28/2
  Dout_CH28/1 -> Manual Switch29/1
  Zero_Dout_CH28/1 -> Manual Switch29/2
  Dout_CH29/1 -> Manual Switch30/1
  Zero_Dout_CH29/1 -> Manual Switch30/2
  Dout_CH30/1 -> Manual Switch31/1
  Zero_Dout_CH30/1 -> Manual Switch31/2
  Dout_CH31/1 -> Manual Switch32/1
  Zero_Dout_CH31/1 -> Manual Switch32/2
  Manual Switch25/1 -> Bus Creator/1  "states 25"
  Manual Switch26/1 -> Bus Creator/2  "states 26"
  Manual Switch27/1 -> Bus Creator/3  "states 27"
  Manual Switch28/1 -> Bus Creator/4  "states 28"
  Manual Switch29/1 -> Bus Creator/5  "states 29"
  Manual Switch30/1 -> Bus Creator/6  "states 30"
  Manual Switch31/1 -> Bus Creator/7  "states 31"
  Manual Switch32/1 -> Bus Creator/8  "states 32"

== system NGGenset_Test_System/SM_Master/Generator/GenSet_4MVA_copy1mva/4MVA Generator with  Primary Controllers/Diesel Engine Speed & Voltage Control fast ==
  note: originally ++
  note: originally ++
  note: These biases may need to
      | go to the references as opposed
      | to the measured signal.
  note: This is the device analog output of =-10Vdc to
      | the HIL Analog Input it should be scaled to 1 pu
  wref : Inport  SampleTime=Ts
  Vtref : Inport  Port=2  SampleTime=Ts
  Generator Enable : Inport  Port=3  SampleTime=Ts
  m : Inport  Port=4  SampleTime=Ts
  w_meas_Wood : Inport  Port=5  SampleTime=Ts
  V_meas_Wood : Inport  Port=6  SampleTime=Ts
  Woodward Enable : Inport  Port=7  SampleTime=Ts
  Bus Creator : BusCreator  Inputs=2
  Bus Creator1 : BusCreator  Inputs=2
  Bus Creator2 : BusCreator  Inputs=2
  Bus Selector : BusSelector  OutputSignals="Mechanical.Rotor speed  wm (pu)"
  Bus Selector1 : BusSelector  OutputSignals="dq0 components.Stator voltage  vd (pu),dq0 components.Stator voltage  vq (pu)"  OutputAsBus=on
  Bus to Vector : BusToVector
  Constant1 : Constant  Value=0
  Constant2 : Constant  Value=0
  Discrete PID Controller1 : simulink/Continuous/PID Controller  Controller=PID  TimeDomain=Discrete-time  SampleTime=-1  IntegratorMethod=Forward Euler  FilterMethod=Forward Euler  Form=Parallel  P=1  I=0  D=0  N=100  InitialConditionSource=internal  InitialConditionForIntegrator=0  InitialConditionForFilter=0  ExternalReset=either  LimitOutput=on  UpperSaturationLimit=5  LowerSaturationLimit=-5  LinearizeAsGain=off  AntiWindupMode=none  Kb=1  TrackingMode=off  Kt=1  PParamMin=[]  PParamMax=[]  IParamMin=[]  IParamMax=[]  DParamMin=[]  DParamMax=[]  NParamMin=[]  NParamMax=[]  KbParamMin=[]  KbParamMax=[]  KtParamMin=[]  KtParamMax=[]  POutMin=[]  POutMax=[]  IOutMin=[]  IOutMax=[]  DOutMin=[]  DOutMax=[]  NOutMin=[]  NOutMax=[]  KbOutMin=[]  KbOutMax=[]  KtOutMin=[]  KtOutMax=[]  IntegratorOutMin=[]  IntegratorOutMax=[]  FilterOutMin=[]  FilterOutMax=[]  SumOutMin=[]  SumOutMax=[]  SumI1OutMin=[]  SumI1OutMax=[]  SumI2OutMin=[]  SumI2OutMax=[]  SumI3OutMin=[]  SumI3OutMax=[]  SumDOutMin=[]  SumDOutMax=[]  SaturationOutMin=[]  SaturationOutMax=[]  IntegratorContinuousStateAttributes=''  IntegratorStateMustResolveToSignalObject=off  IntegratorRTWStateStorageClass=Auto  FilterContinuousStateAttributes=''  FilterStateMustResolveToSignalObject=off  FilterRTWStateStorageClass=Auto
  Excitation : Subsystem  mask(Excitation System){tr=20e-4, reg=[ 200 2e-3 ], exc=[ 1 0.00000001 ], tgr=[ 1e-12 1e-12 ], damp=[0 1e-12 ], sat=[], lim=[ 0 5 0 ], v0=[ 0 0 ]}
      mask prompts: tr "Low-pass filter time constant Tr:"; reg "Regulator gain and time constant [ Ka  Ta ]:"; exc "Exciter  [ Ke  Te ]:"; tgr "Transient gain reduction [ Tb  Tc ]:"; damp "Damping filter gain and time constant  [ Kf  Tf  ]:"; sat "Field saturation parameters [ A B ]:"; lim "Regulator output limits and gain [ Efmin  Efmax  Kp ]:"; v0 "Initial values of terminal voltage  and field voltage [ Vt0 Vf0 ] :"
      mask help:
      | Implements an IEEE type 1 synchronous machine voltage regulator combined
      | to an exciter.
      |
      | The output of the block is the field voltage vfd, in pu,  to be applied to the Vf
      | Simulink input of a Synchronous Machine block.
      |
      | Connect the Vd and Vq measurements signals of the Synchronous Machine block
      | (signals 9 and 10)  to  the Vd and Vq inputs of the Excitation System block.
      mask Help: helpview(psbhelp);
  Fcn1 : Fcn  Expr=sqrt(u(1)^2 + u(2)^2)
  GOVERNOR & DIESEL ENGINE1 : Subsystem  mask(Diesel Engine & Governor){K=10, Ta=[0.025 0.0009 0.00574], Tlim=[0 1.1], Td=0.024, Pm0=0.00005}
      mask prompts: K "Regulator gain K:"; Ta "Actuator time constants [T4 T5 T6] (s) :"; Tlim "Torque limits [Tmin Tmax] (pu) :"; Td "Engine time delay Td (s) :"; Pm0 "Initial value of mechanical power  Pm0 (pu) :"
      mask help:
      | This block implements a diesel engine and governor system:
      | 1st and 2nd inputs: Desired and actual speed (pu)
      | Output: Diesel engine mechanical power.Motor inertia should be combined with generator.
      |
      | Actuator transfer function :
      |      Ha= (1+T4.s) / [ (s (1+T5.s)(1+T6.s) ]
      | Motor :
      |      Time delay Td
      |
      | (See reference in Tutorial Session 5)
  Ground : Ground
  Scope : Scope
      settings: YMin=-5.5  YMax=5.5
  Sum : Sum  Inputs=|++
  Sum1 : Sum  Inputs=|++
  Switch1 : Switch  Threshold=0.5
  Switch2 : Switch  Threshold=0.5
  Pm : Outport
  Vf : Outport  Port=2
  Vt : Outport  Port=3
  w : Outport  Port=4
  Misc : Outport  Port=5
  wires:
  Sum/1 -> GOVERNOR & DIESEL ENGINE1/1(wref (pu))  "wms"
  wref/1 -> Sum/2
  Sum1/1 -> Excitation/1(vref)
  Vtref/1 -> Sum1/2
  Switch2/1 -> Bus Creator1/1, Sum1/1  "wood_AVR_bias"
  Constant1/1 -> Switch2/3
  Constant2/1 -> Switch1/3
  w_meas_Wood/1 -> Switch1/1
  Switch1/1 -> Bus Creator/1, Sum/1  "wood_Gov_bias"
  Woodward Enable/1 -> Switch2/2, Switch1/2
  Bus Creator2/1 -> Misc/1, Scope/1
  Discrete PID Controller1/1 -> Bus Creator2/2, Vf/1  "Vf_after"
  Excitation/1(Vf1) -> Bus Creator2/1, Discrete PID Controller1/1  "Vf_before"
  Bus Creator1/1 -> Vt/1
  Bus Creator/1 -> w/1
  Ground/1 -> Excitation/3(vstab)
  Fcn1/1 -> Excitation/2(v), Bus Creator1/2  "vms"
  V_meas_Wood/1 -> Switch2/1
  Bus Selector/1 -> GOVERNOR & DIESEL ENGINE1/2(w (pu)), Bus Creator/2  "<Rotor speed  wm (pu)>"
  m/1 -> Bus Selector1/1, Bus Selector/1
  Bus Selector1/1 -> Bus to Vector/1
  Bus to Vector/1 -> Fcn1/1
  Generator Enable/1 -> Discrete PID Controller1/2, GOVERNOR & DIESEL ENGINE1/3(Reset)
  GOVERNOR & DIESEL ENGINE1/1(Pmec (pu)) -> Pm/1  "Pmec_gov"

== system NGGenset_Test_System/SM_Master/Generator/GenSet_4MVA_copy1mva/Simulated Generator Controller 3.5 MW/PQ control ==
  P_ref (pu) : Inport
  P (pu) : Inport  Port=2
  Q_ref (pu) : Inport  Port=3
  Q (pu) : Inport  Port=4
  Discrete PID Controller : simulink/Continuous/PID Controller  Controller=PID  TimeDomain=Discrete-time  SampleTime=-1  IntegratorMethod=Forward Euler  FilterMethod=Forward Euler  Form=Parallel  P=0.025  I=1  D=0  N=10  InitialConditionSource=internal  InitialConditionForIntegrator=0  InitialConditionForFilter=0  ExternalReset=none  LimitOutput=on  UpperSaturationLimit=1.15  LowerSaturationLimit=0.85  LinearizeAsGain=off  AntiWindupMode=back-calculation  Kb=1  TrackingMode=off  Kt=1  PParamMin=[]  PParamMax=[]  IParamMin=[]  IParamMax=[]  DParamMin=[]  DParamMax=[]  NParamMin=[]  NParamMax=[]  KbParamMin=[]  KbParamMax=[]  KtParamMin=[]  KtParamMax=[]  POutMin=[]  POutMax=[]  IOutMin=[]  IOutMax=[]  DOutMin=[]  DOutMax=[]  NOutMin=[]  NOutMax=[]  KbOutMin=[]  KbOutMax=[]  KtOutMin=[]  KtOutMax=[]  IntegratorOutMin=[]  IntegratorOutMax=[]  FilterOutMin=[]  FilterOutMax=[]  SumOutMin=[]  SumOutMax=[]  SumI1OutMin=[]  SumI1OutMax=[]  SumI2OutMin=[]  SumI2OutMax=[]  SumI3OutMin=[]  SumI3OutMax=[]  SumDOutMin=[]  SumDOutMax=[]  SaturationOutMin=[]  SaturationOutMax=[]  IntegratorContinuousStateAttributes=''  IntegratorStateMustResolveToSignalObject=off  IntegratorRTWStateStorageClass=Auto  FilterContinuousStateAttributes=''  FilterStateMustResolveToSignalObject=off  FilterRTWStateStorageClass=Auto
  Discrete PID Controller1 : simulink/Continuous/PID Controller  Controller=PID  TimeDomain=Discrete-time  SampleTime=-1  IntegratorMethod=Forward Euler  FilterMethod=Forward Euler  Form=Parallel  P=0.2  I=1.5  D=0  N=10  InitialConditionSource=internal  InitialConditionForIntegrator=0  InitialConditionForFilter=0  ExternalReset=none  LimitOutput=on  UpperSaturationLimit=1.15  LowerSaturationLimit=0.85  LinearizeAsGain=off  AntiWindupMode=back-calculation  Kb=1  TrackingMode=off  Kt=1  PParamMin=[]  PParamMax=[]  IParamMin=[]  IParamMax=[]  DParamMin=[]  DParamMax=[]  NParamMin=[]  NParamMax=[]  KbParamMin=[]  KbParamMax=[]  KtParamMin=[]  KtParamMax=[]  POutMin=[]  POutMax=[]  IOutMin=[]  IOutMax=[]  DOutMin=[]  DOutMax=[]  NOutMin=[]  NOutMax=[]  KbOutMin=[]  KbOutMax=[]  KtOutMin=[]  KtOutMax=[]  IntegratorOutMin=[]  IntegratorOutMax=[]  FilterOutMin=[]  FilterOutMax=[]  SumOutMin=[]  SumOutMax=[]  SumI1OutMin=[]  SumI1OutMax=[]  SumI2OutMin=[]  SumI2OutMax=[]  SumI3OutMin=[]  SumI3OutMax=[]  SumDOutMin=[]  SumDOutMax=[]  SaturationOutMin=[]  SaturationOutMax=[]  IntegratorContinuousStateAttributes=''  IntegratorStateMustResolveToSignalObject=off  IntegratorRTWStateStorageClass=Auto  FilterContinuousStateAttributes=''  FilterStateMustResolveToSignalObject=off  FilterRTWStateStorageClass=Auto
  Sum : Sum  Inputs=|-+
  Sum1 : Sum  Inputs=|-+
  w_ref (pu) : Outport
  V_ref (pu) : Outport  Port=2
  wires:
  Q_ref (pu)/1 -> Sum1/2  "ref"
  Discrete PID Controller1/1 -> V_ref (pu)/1  "v"
  Q (pu)/1 -> Sum1/1  "pu"
  Sum1/1 -> Discrete PID Controller1/1  "dq"
  P_ref (pu)/1 -> Sum/2
  Discrete PID Controller/1 -> w_ref (pu)/1
  P (pu)/1 -> Sum/1
  Sum/1 -> Discrete PID Controller/1

== system NGGenset_Test_System/SM_Master/Generator/GenSet_4MVA_copy1mva/Simulated Generator Controller 3.5 MW/PV control ==
  P_ref (pu) : Inport
  P (pu) : Inport  Port=2
  Discrete PID Controller : simulink/Continuous/PID Controller  Controller=PID  TimeDomain=Discrete-time  SampleTime=-1  IntegratorMethod=Forward Euler  FilterMethod=Forward Euler  Form=Parallel  P=0.025  I=1  D=0  N=10  InitialConditionSource=internal  InitialConditionForIntegrator=0  InitialConditionForFilter=0  ExternalReset=none  LimitOutput=on  UpperSaturationLimit=1.15  LowerSaturationLimit=0.85  LinearizeAsGain=off  AntiWindupMode=back-calculation  Kb=1  TrackingMode=off  Kt=1  PParamMin=[]  PParamMax=[]  IParamMin=[]  IParamMax=[]  DParamMin=[]  DParamMax=[]  NParamMin=[]  NParamMax=[]  KbParamMin=[]  KbParamMax=[]  KtParamMin=[]  KtParamMax=[]  POutMin=[]  POutMax=[]  IOutMin=[]  IOutMax=[]  DOutMin=[]  DOutMax=[]  NOutMin=[]  NOutMax=[]  KbOutMin=[]  KbOutMax=[]  KtOutMin=[]  KtOutMax=[]  IntegratorOutMin=[]  IntegratorOutMax=[]  FilterOutMin=[]  FilterOutMax=[]  SumOutMin=[]  SumOutMax=[]  SumI1OutMin=[]  SumI1OutMax=[]  SumI2OutMin=[]  SumI2OutMax=[]  SumI3OutMin=[]  SumI3OutMax=[]  SumDOutMin=[]  SumDOutMax=[]  SaturationOutMin=[]  SaturationOutMax=[]  IntegratorContinuousStateAttributes=''  IntegratorStateMustResolveToSignalObject=off  IntegratorRTWStateStorageClass=Auto  FilterContinuousStateAttributes=''  FilterStateMustResolveToSignalObject=off  FilterRTWStateStorageClass=Auto
  Sum : Sum  Inputs=|-+
  w_ref (pu) : Outport
  wires:
  Sum/1 -> Discrete PID Controller/1
  P (pu)/1 -> Sum/1
  Discrete PID Controller/1 -> w_ref (pu)/1
  P_ref (pu)/1 -> Sum/2

== system NGGenset_Test_System/SM_Master/Generator/NG GenSet_3.5MVA_09212015/3.5MVA Generator with  Primary Controllers1/NG Engine Speed & Voltage Control fast ==
  note: originally ++
  note: originally ++
  note: These biases may need to
      | go to the references as opposed
      | to the measured signal.
  note: This is the device analog output of =-10Vdc to
      | the HIL Analog Input it should be scaled to 1 pu
  wref : Inport  SampleTime=Ts
  Vtref : Inport  Port=2  SampleTime=Ts
  Generator Enable : Inport  Port=3  SampleTime=Ts
  m : Inport  Port=4  SampleTime=Ts
  w_meas_Wood : Inport  Port=5  SampleTime=Ts
  V_meas_Wood : Inport  Port=6  SampleTime=Ts
  Woodward Enable : Inport  Port=7  SampleTime=Ts
  Bus Creator : BusCreator  Inputs=2
  Bus Creator1 : BusCreator  Inputs=2
  Bus Creator2 : BusCreator  Inputs=2
  Bus Selector : BusSelector  OutputSignals="Mechanical.Rotor speed  wm (pu)"
  Bus Selector1 : BusSelector  OutputSignals="dq0 components.Stator voltage  vd (pu),dq0 components.Stator voltage  vq (pu)"  OutputAsBus=on
  Bus to Vector : BusToVector
  Constant1 : Constant  Value=0
  Constant2 : Constant  Value=0
  Discrete PID Controller1 : simulink/Continuous/PID Controller  Controller=PID  TimeDomain=Discrete-time  SampleTime=-1  IntegratorMethod=Forward Euler  FilterMethod=Forward Euler  Form=Parallel  P=1  I=0  D=0  N=100  InitialConditionSource=internal  InitialConditionForIntegrator=0  InitialConditionForFilter=0  ExternalReset=either  LimitOutput=on  UpperSaturationLimit=5  LowerSaturationLimit=-5  LinearizeAsGain=off  AntiWindupMode=none  Kb=1  TrackingMode=off  Kt=1  PParamMin=[]  PParamMax=[]  IParamMin=[]  IParamMax=[]  DParamMin=[]  DParamMax=[]  NParamMin=[]  NParamMax=[]  KbParamMin=[]  KbParamMax=[]  KtParamMin=[]  KtParamMax=[]  POutMin=[]  POutMax=[]  IOutMin=[]  IOutMax=[]  DOutMin=[]  DOutMax=[]  NOutMin=[]  NOutMax=[]  KbOutMin=[]  KbOutMax=[]  KtOutMin=[]  KtOutMax=[]  IntegratorOutMin=[]  IntegratorOutMax=[]  FilterOutMin=[]  FilterOutMax=[]  SumOutMin=[]  SumOutMax=[]  SumI1OutMin=[]  SumI1OutMax=[]  SumI2OutMin=[]  SumI2OutMax=[]  SumI3OutMin=[]  SumI3OutMax=[]  SumDOutMin=[]  SumDOutMax=[]  SaturationOutMin=[]  SaturationOutMax=[]  IntegratorContinuousStateAttributes=''  IntegratorStateMustResolveToSignalObject=off  IntegratorRTWStateStorageClass=Auto  FilterContinuousStateAttributes=''  FilterStateMustResolveToSignalObject=off  FilterRTWStateStorageClass=Auto
  Excitation : Subsystem  mask(Excitation System){tr=20e-4, reg=[ 200 2e-3 ], exc=[ 1 0.00000001 ], tgr=[ 1e-12 1e-12 ], damp=[0 1e-12 ], sat=[], lim=[ 0 5 0 ], v0=[ 0 0 ]}
      mask prompts: tr "Low-pass filter time constant Tr:"; reg "Regulator gain and time constant [ Ka  Ta ]:"; exc "Exciter  [ Ke  Te ]:"; tgr "Transient gain reduction [ Tb  Tc ]:"; damp "Damping filter gain and time constant  [ Kf  Tf  ]:"; sat "Field saturation parameters [ A B ]:"; lim "Regulator output limits and gain [ Efmin  Efmax  Kp ]:"; v0 "Initial values of terminal voltage  and field voltage [ Vt0 Vf0 ] :"
      mask help:
      | Implements an IEEE type 1 synchronous machine voltage regulator combined
      | to an exciter.
      |
      | The output of the block is the field voltage vfd, in pu,  to be applied to the Vf
      | Simulink input of a Synchronous Machine block.
      |
      | Connect the Vd and Vq measurements signals of the Synchronous Machine block
      | (signals 9 and 10)  to  the Vd and Vq inputs of the Excitation System block.
      mask Help: helpview(psbhelp);
  Fcn1 : Fcn  Expr=sqrt(u(1)^2 + u(2)^2)
  GE/Jenbacher J620 NG Engine (1800 RPM)1 : Subsystem  mask{cd=.8, H=47133, keq=1.3962, Ma=.029, Meq=.0285, Mf=.019, P0=800000, Pm=37241, R=8.314, T0=300, Tm=325, thermalEfficiency=.45, V=0.031, Vd=0.125, volumeEfficiency=.9, P=3, I=3, UL=1.05, LL=0, UPL=1.5, LPL=-1.5}
      mask prompts: cd "Discharge coefficient - cd"; H "NG heating value - H"; keq "Equivalent ratio of specific heats of air/fuel mixture - keq"; Ma "Molecular weight of air - Ma"; Meq "Equivalent molecular weight of air/fuel mixture - Meq"; Mf "Molecular weight of NG - Mf"; P0 "Throttle inlet air pressure - P0"; Pm "Intake manifold pressure - Pm"; R "Universal gas constant - R"; T0 "Throttle inlet charge temperature - T0"; Tm "Intake manifold temperature - Tm"; thermalEfficiency "Thermal efficiency - thermalEfficiency"; V "Manifold plus port passage volume - V"; Vd "Engine displacement - Vd"; volumeEfficiency "Volumetric efficiency - volumeEfficiency"; P "Proportional Gain - P"; I "Integral Gain - I"; UL "Upper Integrator Limit - UL"; LL "Lower Integrator Limit - LL"; UPL "Upper Power Limit - UPL"; LPL "Lower Power Limit - LPL"
      mask help: All units are MKS. Refer to "Modeling and Validation of a Lean Burn Natural Gas Engine", Gangopadhyay et. al., ASME 2001
  Ground : Ground
  Sum : Sum  Inputs=|++
  Sum1 : Sum  Inputs=|++
  Switch1 : Switch  Threshold=0.5
  Switch2 : Switch  Threshold=0.5
  Pm : Outport
  Vf : Outport  Port=2
  Vt : Outport  Port=3
  w : Outport  Port=4
  Misc : Outport  Port=5
  Themal data : Outport  Port=6
  wires:
  Sum/1 -> GE/Jenbacher J620 NG Engine (1800 RPM)1/1(wref (pu))  "wms"
  wref/1 -> Sum/2
  Sum1/1 -> Excitation/1(vref)
  Vtref/1 -> Sum1/2
  Switch2/1 -> Sum1/1, Bus Creator1/1  "wood_AVR_bias"
  Constant1/1 -> Switch2/3
  Constant2/1 -> Switch1/3
  w_meas_Wood/1 -> Switch1/1
  Switch1/1 -> Bus Creator/1, Sum/1  "wood_Gov_bias"
  Woodward Enable/1 -> Switch2/2, Switch1/2
  Bus Creator2/1 -> Misc/1
  Discrete PID Controller1/1 -> Bus Creator2/2, Vf/1  "Vf_after"
  Excitation/1(Vf1) -> Bus Creator2/1, Discrete PID Controller1/1  "Vf_before"
  Bus Creator1/1 -> Vt/1
  Bus Creator/1 -> w/1
  Ground/1 -> Excitation/3(vstab)
  Fcn1/1 -> Excitation/2(v), Bus Creator1/2  "vms"
  V_meas_Wood/1 -> Switch2/1
  Bus Selector/1 -> GE/Jenbacher J620 NG Engine (1800 RPM)1/2(w (pu)), Bus Creator/2  "<Rotor speed  wm (pu)>"
  m/1 -> Bus Selector1/1, Bus Selector/1
  Bus Selector1/1 -> Bus to Vector/1
  Bus to Vector/1 -> Fcn1/1
  Generator Enable/1 -> GE/Jenbacher J620 NG Engine (1800 RPM)1/3("Reset if both \"Gen Starter\" and \"Gen Fuel\" are low"), Discrete PID Controller1/2
  GE/Jenbacher J620 NG Engine (1800 RPM)1/1(Pmech pu) -> Pm/1  "Pmec_gov"
  GE/Jenbacher J620 NG Engine (1800 RPM)1/2(Thermal Data) -> Themal data/1

== system NGGenset_Test_System/SM_Master/Generator/NG GenSet_3.5MVA_09212015/Simulated Generator Controller 3.5 MW/PQ control ==
  P_ref (pu) : Inport
  P (pu) : Inport  Port=2
  Q_ref (pu) : Inport  Port=3
  Q (pu) : Inport  Port=4
  Discrete PID Controller : simulink/Continuous/PID Controller  Controller=PID  TimeDomain=Discrete-time  SampleTime=-1  IntegratorMethod=Forward Euler  FilterMethod=Forward Euler  Form=Parallel  P=0.025  I=1  D=0  N=10  InitialConditionSource=internal  InitialConditionForIntegrator=0  InitialConditionForFilter=0  ExternalReset=none  LimitOutput=on  UpperSaturationLimit=1.15  LowerSaturationLimit=0.85  LinearizeAsGain=off  AntiWindupMode=back-calculation  Kb=1  TrackingMode=off  Kt=1  PParamMin=[]  PParamMax=[]  IParamMin=[]  IParamMax=[]  DParamMin=[]  DParamMax=[]  NParamMin=[]  NParamMax=[]  KbParamMin=[]  KbParamMax=[]  KtParamMin=[]  KtParamMax=[]  POutMin=[]  POutMax=[]  IOutMin=[]  IOutMax=[]  DOutMin=[]  DOutMax=[]  NOutMin=[]  NOutMax=[]  KbOutMin=[]  KbOutMax=[]  KtOutMin=[]  KtOutMax=[]  IntegratorOutMin=[]  IntegratorOutMax=[]  FilterOutMin=[]  FilterOutMax=[]  SumOutMin=[]  SumOutMax=[]  SumI1OutMin=[]  SumI1OutMax=[]  SumI2OutMin=[]  SumI2OutMax=[]  SumI3OutMin=[]  SumI3OutMax=[]  SumDOutMin=[]  SumDOutMax=[]  SaturationOutMin=[]  SaturationOutMax=[]  IntegratorContinuousStateAttributes=''  IntegratorStateMustResolveToSignalObject=off  IntegratorRTWStateStorageClass=Auto  FilterContinuousStateAttributes=''  FilterStateMustResolveToSignalObject=off  FilterRTWStateStorageClass=Auto
  Discrete PID Controller1 : simulink/Continuous/PID Controller  Controller=PID  TimeDomain=Discrete-time  SampleTime=-1  IntegratorMethod=Forward Euler  FilterMethod=Forward Euler  Form=Parallel  P=0.2  I=1.5  D=0  N=10  InitialConditionSource=internal  InitialConditionForIntegrator=0  InitialConditionForFilter=0  ExternalReset=none  LimitOutput=on  UpperSaturationLimit=1.15  LowerSaturationLimit=0.85  LinearizeAsGain=off  AntiWindupMode=back-calculation  Kb=1  TrackingMode=off  Kt=1  PParamMin=[]  PParamMax=[]  IParamMin=[]  IParamMax=[]  DParamMin=[]  DParamMax=[]  NParamMin=[]  NParamMax=[]  KbParamMin=[]  KbParamMax=[]  KtParamMin=[]  KtParamMax=[]  POutMin=[]  POutMax=[]  IOutMin=[]  IOutMax=[]  DOutMin=[]  DOutMax=[]  NOutMin=[]  NOutMax=[]  KbOutMin=[]  KbOutMax=[]  KtOutMin=[]  KtOutMax=[]  IntegratorOutMin=[]  IntegratorOutMax=[]  FilterOutMin=[]  FilterOutMax=[]  SumOutMin=[]  SumOutMax=[]  SumI1OutMin=[]  SumI1OutMax=[]  SumI2OutMin=[]  SumI2OutMax=[]  SumI3OutMin=[]  SumI3OutMax=[]  SumDOutMin=[]  SumDOutMax=[]  SaturationOutMin=[]  SaturationOutMax=[]  IntegratorContinuousStateAttributes=''  IntegratorStateMustResolveToSignalObject=off  IntegratorRTWStateStorageClass=Auto  FilterContinuousStateAttributes=''  FilterStateMustResolveToSignalObject=off  FilterRTWStateStorageClass=Auto
  Sum : Sum  Inputs=|-+
  Sum1 : Sum  Inputs=|-+
  w_ref (pu) : Outport
  V_ref (pu) : Outport  Port=2
  wires:
  Sum/1 -> Discrete PID Controller/1
  P (pu)/1 -> Sum/1
  Discrete PID Controller/1 -> w_ref (pu)/1
  P_ref (pu)/1 -> Sum/2
  Sum1/1 -> Discrete PID Controller1/1  "dq"
  Q (pu)/1 -> Sum1/1  "pu"
  Discrete PID Controller1/1 -> V_ref (pu)/1  "v"
  Q_ref (pu)/1 -> Sum1/2  "ref"

== system NGGenset_Test_System/SM_Master/Generator/NG GenSet_3.5MVA_09212015/Simulated Generator Controller 3.5 MW/PV control ==
  P_ref (pu) : Inport
  P (pu) : Inport  Port=2
  Discrete PID Controller : simulink/Continuous/PID Controller  Controller=PID  TimeDomain=Discrete-time  SampleTime=-1  IntegratorMethod=Forward Euler  FilterMethod=Forward Euler  Form=Parallel  P=0.025  I=1  D=0  N=10  InitialConditionSource=internal  InitialConditionForIntegrator=0  InitialConditionForFilter=0  ExternalReset=none  LimitOutput=on  UpperSaturationLimit=1.15  LowerSaturationLimit=0.85  LinearizeAsGain=off  AntiWindupMode=back-calculation  Kb=1  TrackingMode=off  Kt=1  PParamMin=[]  PParamMax=[]  IParamMin=[]  IParamMax=[]  DParamMin=[]  DParamMax=[]  NParamMin=[]  NParamMax=[]  KbParamMin=[]  KbParamMax=[]  KtParamMin=[]  KtParamMax=[]  POutMin=[]  POutMax=[]  IOutMin=[]  IOutMax=[]  DOutMin=[]  DOutMax=[]  NOutMin=[]  NOutMax=[]  KbOutMin=[]  KbOutMax=[]  KtOutMin=[]  KtOutMax=[]  IntegratorOutMin=[]  IntegratorOutMax=[]  FilterOutMin=[]  FilterOutMax=[]  SumOutMin=[]  SumOutMax=[]  SumI1OutMin=[]  SumI1OutMax=[]  SumI2OutMin=[]  SumI2OutMax=[]  SumI3OutMin=[]  SumI3OutMax=[]  SumDOutMin=[]  SumDOutMax=[]  SaturationOutMin=[]  SaturationOutMax=[]  IntegratorContinuousStateAttributes=''  IntegratorStateMustResolveToSignalObject=off  IntegratorRTWStateStorageClass=Auto  FilterContinuousStateAttributes=''  FilterStateMustResolveToSignalObject=off  FilterRTWStateStorageClass=Auto
  Sum : Sum  Inputs=|-+
  w_ref (pu) : Outport
  wires:
  P_ref (pu)/1 -> Sum/2
  Discrete PID Controller/1 -> w_ref (pu)/1
  P (pu)/1 -> Sum/1
  Sum/1 -> Discrete PID Controller/1
